simulink model "on_line2"  (R2018a)
settings: Solver=VariableStepAuto  StartTime=0.0  StopTime=20  RelTol=1e-3
libraries: ctrlSharedLib x1
settings Model: Creator=Dominik  LastModifiedBy=Dominik

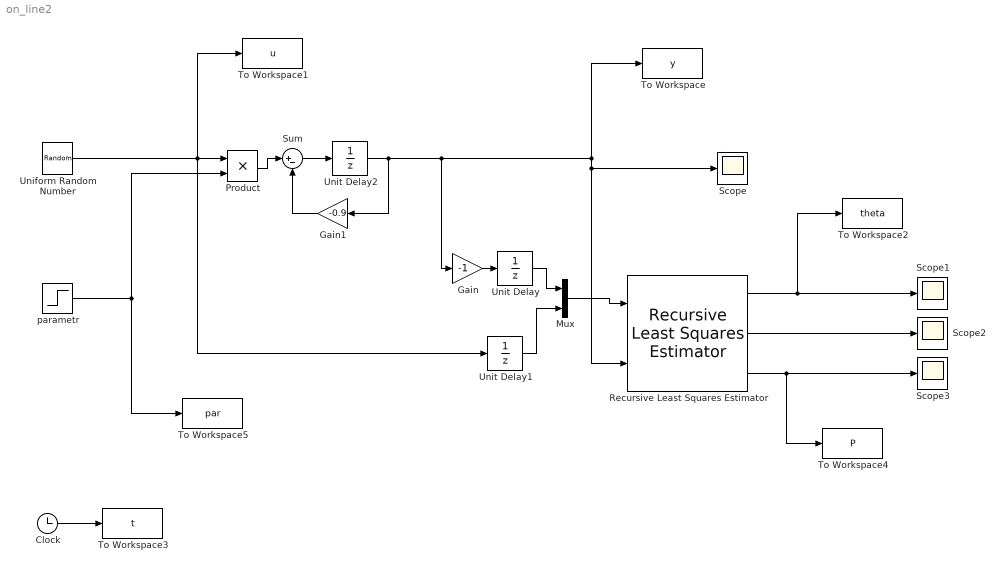
== system on_line2 ==
  Clock : Clock
  Gain : Gain  Gain=-1
  Gain1 : Gain  Gain=-0.9
  Mux : Mux  Inputs=2
  Product : Product
  Recursive Least Squares Estimator : ctrlSharedLib/Recursive Least Squares Estimator  InitialEstimateSource=None  InitialParameterData=2  P0=100  EstimationMethod=Forgetting Factor  AdaptationParameter=0.95  HasTimeVaryingAdaptationParameter=off  NormalizationBias=eps  OutputError=on  OutputP=on  AddEnablePort=off  Ts=-1
      settings: SourceProductName=Control System Toolbox  SourceProductBaseCode=CT
  Scope{,1..3} (4 alike) : Scope
  Sum : Sum  Inputs=|+-
  To Workspace : ToWorkspace  VariableName=y  SampleTime=-1
  To Workspace1 : ToWorkspace  VariableName=u  SampleTime=-1
  To Workspace2 : ToWorkspace  VariableName=theta  SampleTime=-1
  To Workspace3 : ToWorkspace  VariableName=t  SampleTime=-1
  To Workspace4 : ToWorkspace  VariableName=P  SampleTime=-1
  To Workspace5 : ToWorkspace  VariableName=par  SampleTime=-1
  Uniform Random Number : UniformRandomNumber  SampleTime=0.1
  Unit Delay : UnitDelay  SampleTime=-1
  Unit Delay1 : UnitDelay  SampleTime=-1
  Unit Delay2 : UnitDelay  SampleTime=-1
  parametr : Step  Time=10  Before=0.2  After=0.4  SampleTime=0
  wires:
  Unit Delay2/1 -> Gain1/1, Scope/1, Recursive Least Squares Estimator/2, To Workspace/1, Gain/1
  Gain/1 -> Unit Delay/1
  Unit Delay/1 -> Mux/1
  Unit Delay1/1 -> Mux/2
  Uniform Random Number/1 -> Product/1, To Workspace1/1, Unit Delay1/1
  Mux/1 -> Recursive Least Squares Estimator/1
  Recursive Least Squares Estimator/1 -> To Workspace2/1, Scope1/1
  Clock/1 -> To Workspace3/1
  Recursive Least Squares Estimator/2 -> Scope2/1
  Recursive Least Squares Estimator/3 -> To Workspace4/1, Scope3/1
  Sum/1 -> Unit Delay2/1
  parametr/1 -> To Workspace5/1, Product/2
  Product/1 -> Sum/1
  Gain1/1 -> Sum/2
